simulink subsystem "ActiveDifferential2"  (R2024a)
settings: Solver=VariableStepAuto  StartTime=0.0  StopTime=10.0  RelTol=1e-3
libraries: autolibshareddiff x1
settings Model: Creator=The MathWorks, Inc.  LastModifiedBy=The MathWorks, Inc.
settings RTWCC: GPUComputeCapability=3.5

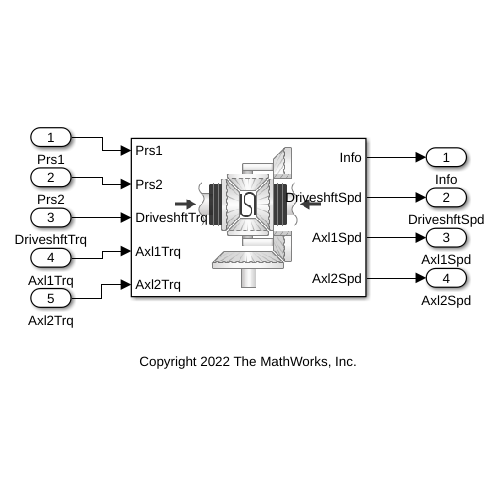
[thumbnail: Simulink's stored preview of the top-level diagram]
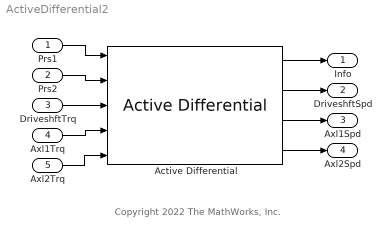
== system ActiveDifferential2 ==
  note: Copyright 2022 The MathWorks, Inc.
  Prs1 : Inport
  Prs2 : Inport  Port=2
  DriveshftTrq : Inport  Port=3
  Axl1Trq : Inport  Port=4
  Axl2Trq : Inport  Port=5
  Active Differential : autolibshareddiff/Active Differential  VariantControl=Active Differential  diffType=Spur gears, superposition clutches  Ns1=PlntDiffrntl2Cltch1CaseGearRatio  Ns2=PlntDiffrntl2Cltch2CaseGearRatio  Jgc=PlntDiffrntl2ThreeGangGearInertia  Np1=PlntDiffrntl2CltchAxl1CarrGearRatio  Js1=PlntDiffrntl2CltchAxl1SunGearInertia  Jc1=PlntDiffrntl2CltchAxl1CarrInertia  Jr1=PlntDiffrntl2CltchAxl1RingInertia  Np2=PlntDiffrntl2CltchAxl2CarrGearRatio  Js2=PlntDiffrntl2CltchAxl2SunGearInertia  Jc2=PlntDiffrntl2CltchAxl2CarrInertia  Jr2=PlntDiffrntl2CltchAxl2RingInertia  shaftSwitchMask=To the left of center-line  Ndiff=PlntDiffrntl2Ratio  Jd=PlntDiffrntl2CarrInertia  bd=PlntDiffrntl2CarrDamp  Jw1=PlntDiffrntl2Axl1Inertia  bw1=PlntDiffrntl2Axl1Damp  Jw2=PlntDiffrntl2Axl2Inertia  bw2=PlntDiffrntl2Axl2Damp  omegaw1o=PlntDiffrntl2Axl1InitVel  omegaw2o=PlntDiffrntl2Axl2InitVel  couplingType=Pre-loaded ideal clutch  Aeff=PlntDiffrntl2CltchAppPrsArea  Ndisks=PlntDiffrntl2CltchNumDisk  Reff=PlntDiffrntl2CltchRadius  Fc=PlntDiffrntl2CltchPreloadForce  muc=PlntDiffrntl2CltchFricVect  dw=PlntDiffrntl2CltchSpdVect  TdPdw=PlntDiffrntl2CltchTrqSlipSpdVect  pT=PlntDiffrntl2CltchPrsVect  dwT=PlntDiffrntl2CltchSlipSpdVect  tauC=PlntDiffrntl2CltchCplngTimeCnst  IdealInterpMethod=Linear point-slope  IdealExtrapMethod=Clip  TdwInterpMethod=Linear point-slope  TdwExtrapMethod=Clip  maxAbsSpd=5e3  aMode=6  blkID=0
  Info : Outport
  DriveshftSpd : Outport  Port=2
  Axl1Spd : Outport  Port=3
  Axl2Spd : Outport  Port=4
  wires:
  Active Differential/1 -> Info/1
  Active Differential/2 -> DriveshftSpd/1
  Active Differential/3 -> Axl1Spd/1
  Active Differential/4 -> Axl2Spd/1
  DriveshftTrq/1 -> Active Differential/3
  Axl2Trq/1 -> Active Differential/5
  Axl1Trq/1 -> Active Differential/4
  Prs2/1 -> Active Differential/2
  Prs1/1 -> Active Differential/1
